simulink library "sm_car_lib_more_examples"  (R2025a)
settings: Solver=VariableStepAuto  StartTime=0.0  StopTime=10.0  RelTol=1e-3
undefined symbols (not defined in the file or in its folder): Linkage, Right, UAc, UAf, UAr, Visual, VisualVisual, X, Y, Z
libraries: sm_lib x109, Suspension_Utilities x45, fl_lib x4, nesl_utility x2
(part 1 of 6)
Description:
  | Copyright 2020-2025 The MathWorks, Inc.
settings Model: Creator=smiller  LastModifiedBy=smiller
settings SolverCC: AlgebraicLoopSolver=TrustRegion
settings DataIOCC: ReturnWorkspaceOutputs=off
settings OptimizationCC: ReuseModelBlockBuffer=off
settings DebuggingCC: UnconnectedInputMsg=warning  UnconnectedOutputMsg=warning  UnconnectedLineMsg=warning  ArithmeticOperatorsInVariantConditions=warning
settings ModelReferenceCC: EnableRefExpFcnMdlSchedulingChecks=on
settings SFSimCC: CustomCodeUndefinedFunction=UseInterfaceOnly
settings RTWCC: GPUComputeCapability=3.5

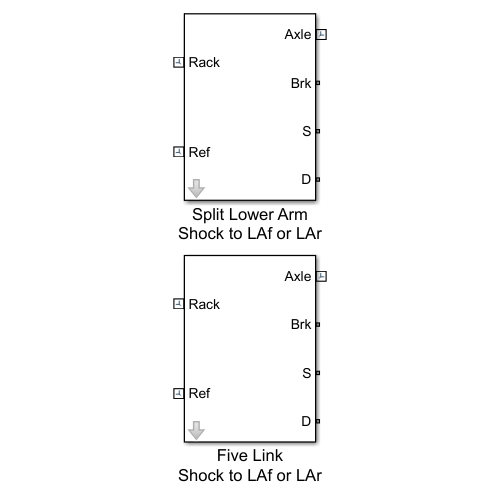
[thumbnail: Simulink's stored preview of the top-level diagram]
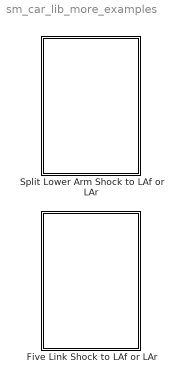
== system sm_car_lib_more_examples ==
  Five Link Shock to LAf or LAr : Subsystem  VariantControl=Link5_StoLAFoR  mask(Five-Link Suspension, Shock to Rear){popup_leftRight=Right, hp_in_f_ua=Linkage.Upper_Arm.HPInboardF.Value, hp_in_r_ua=Linkage.Upper_Arm.HPInboardR.Value, hp_out_f_ua=Linkage.Upper_Arm.HPOutboardF.Value, hp_out_r_ua=Linkage.Upper_Arm.HPOutboardR.Value, hp_in_f_la=Linkage.Lower_Arm.HPInboardF.Value, hp_in_r_la=Linkage.Lower_Arm.HPInboardR.Value, hp_out_f_la=Linkage.Lower_Arm.HPOutboardF.Value, hp_out_r_la=Linkage.Lower_Arm.HPOutboardR.Value, hp_upr_cg=Linkage.Upright.HPCG.Value, hp_upr_wc=Linkage.Upright.HPWheelCtr.Value, hp_in_rod=Linkage.Track_Rod.HPInboard.Value, hp_upr_rod=Linkage.Track_Rod.HPOutboard.Value, hp_spr_top=Linkage.Spring.HPTop.Value, hp_spr_bot=Linkage.Spring.HPBottom.Value, clr_hp=Visual.hp.clr, opc_hp=Visual.hp.opc, size_hp=Visual.hp.rad, uaf_mass=Linkage.Upper_Arm.Mass.Value, uar_mass=Linkage.Upper_Arm.Mass.Value, laf_mass=Linkage.Lower_Arm.Mass.Value, lar_mass=Linkage.Lower_Arm.Mass.Value, clr_conn_links=Visual.hp.clr, opc_conn_links=Visual.hp.opc, size_conn_links=Visual.hp.rad, clr_uaf=Visual.UpperArm.clr, opc_uaf=Visual.part.opc, radius_uaf=Visual.UpperArm.rad, clr_uar=Visual.UpperArm.clr, opc_uar=Visual.part.opc, radius_uar=Visual.UpperArm.rad, clr_laf=Visual.LowerArm.clr, opc_laf=Visual.part.opc, radius_laf=Visual.LowerArm.clr, clr_lar=Visual.LowerArm.clr, opc_lar=Visual.part.opc, radius_lar=Visual.LowerArm.rad, spr_la_att=Linkage.Spring.class.Value, shock_pist_mass=Linkage.Piston.Mass.Value, shock_cyl_mass=Linkage.Cylinder.Mass.Value, up_lim_bumpstop=Linkage.Bumpstops.Upper_Limit.Value, low_lim_bumpstop=Linkage.Bumpstops.Lower_Limit.Value, clr_conn_shock=Visual.hp.clr, opc_conn_shock=Visual.hp.opc, size_conn_shock=Visual.hp.rad, clr_shock_cyl=Visual.Shock.cyl.clr, opc_shock_cyl=Visual.part.opc, radius_shock_cyl=Visual.Shock.cyl.rad, clr_shock_piston=Visual.Shock.piston.clr, opc_shock_piston=Visual.part.opc, clr_shock_bumpstop=Visual.Shock.bumpstop.clr, opc_shock_bumpstop=Visual.part.opc, deadvol_len_shock_cyl=Visual.Shock.dead_length, piston_len_shock=Visual.Shock.piston.len, cyl_cap_len_shock=Visual.Shock.cap.len, bumpstop_len_shock=Visual.Shock.bumpstop.len, atoe=Linkage.Upright.aToe.Value, acamber=Linkage.Upright.aCamber.Value, upr_mass=Linkage.Upright.Mass.Value, clr_conn_upr=Visual.hp.clr, opc_conn_upr=Visual.hp.opc, size_conn_upr=Visual.hp.rad, clr_upr=Visual.Upright.clr, opc_upr=Visual.part.opc, radius_upr=Visual.Upright.clr, clr_stub_axle=Visual.Axle.clr, opc_stub_axle=Visual.part.opc, radius_stub_axle=Visual.Axle.rad, rod_mass=Linkage.Track_Rod.Mass.Value, clr_conn_rod=Visual.hp.clr, opc_conn_rod=Visual.hp.opc, size_conn_rod=Visual.hp.rad, clr_rod=Visual.TrackRod.clr, opc_rod=Visual.part.opc, radius_rod=Visual.TrackRod.rad, whl_spd_init=Linkage.Upright.Initial_Wheel_Speed.Value}
      mask prompts: popup_leftRight "Left/Right"; hp_in_f_ua "Upper Arm Front [xyz] (m)"; hp_in_r_ua "Upper Arm Rear [xyz] (m)"; hp_out_f_ua "Upper Arm Front Outboard [xyz] (m)"; hp_out_r_ua "Upper Arm Rear Outboard [xyz] (m)"; hp_in_f_la "Lower Arm Front [xyz] (m)"; hp_in_r_la "Lower Arm Rear [xyz] (m)"; hp_out_f_la "Lower Arm Front Outboard [xyz] (m)"; hp_out_r_la "Lower Arm Rear Outboard [xyz] (m)"; hp_upr_cg "Upright CG [xyz] (m)"; hp_upr_wc "Wheel Center [xyz] (m)"; hp_in_rod "Track Rod Inboard [xyz] (m)"; hp_upr_rod "Track Rod Outboard [xyz] (m)"; hp_spr_top "Spring Top [xyz] (m)"; hp_spr_bot "Spring Bottom [xyz] (m)"; spr_la_att "Lower Arm Attach (Front/Rear)"; shock_pist_mass "Piston Mass (kg)"; shock_cyl_mass "Cylinder Mass (kg)"; up_lim_bumpstop "Upper Limit (m)"; low_lim_bumpstop "Lower Limit (m)"; deadvol_len_shock_cyl "Dead Volume Height (m)"; piston_len_shock "Piston Length (m)"; cyl_cap_len_shock "Cylinder Cap Length (m)"; bumpstop_len_shock "Bumpstop Length (m)"; atoe "Toe Angle (deg)"; acamber "Camber Angle (deg)"; upr_mass "Mass (kg)"; rod_mass "Mass (kg)"; whl_spd_init "Initial Wheel Speed (rad/s)"
      mask help: This models a multi-link suspension for steered and non-steered configurations. The non-steered configuration maintains its orientation via the track rods that connect to fixed points on the subframe. The shock absorber connects the subframe and lower rear control arm.
      mask init:
      | if(popup_leftRight == 1)
      |     rhs_susp = 1;
      |     set_param([gcb '/Spring Arm/Front/Arm'],'popup_leftRight','Left');
      |     set_param([gcb '/Spring Arm/Rear/Arm'],'popup_leftRight','Left');
      | elseif(popup_leftRight == 2)
      |     rhs_susp = -1;
      |     set_param([gcb '/Spring Arm/Front/Arm'],'popup_leftRight','Right');
      |     set_param([gcb '/Spring Arm/Rear/Arm'],'popup_leftRight','Right');
      | end
      | 
      | if(strcmpi(spr_la_att,'front'))
      |     set_param([gcb '/Spring Arm'],'LabelModeActiveChoice','Front');
      | elseif(strcmpi(spr_la_att,'rear'))
      |     set_param([gcb '/Spring Arm'],'LabelModeActiveChoice','Rear');
      | end
      mask Help: web('sm_car_double_wishbone_suspension_help.html')
      mask TypeOptions popup_leftRight:
      | Hardpoints/popup_leftRight | Upright/popup_leftRight | Lower Arm Rear/popup_leftRight | Lower Arm Front/popup_leftRight | Track Rod/popup_leftRight | Upper Arm Front/popup_leftRight | Upper Arm Rear/popup_leftRight | Universal
      | HP LAF/popup_leftRight | Universal
      | HP LAR/popup_leftRight | Universal
      | HP UAF/popup_leftRight | Universal
      | HP UAR/popup_leftRight
      mask TypeOptions hp_in_f_ua:
      | Hardpoints/hp_in_f_ua | Upper Arm Front/hp_in | Universal
      | HP UAF/hp_f | Universal
      | HP UAR/hp_f
      mask TypeOptions hp_in_r_ua:
      | Hardpoints/hp_in_r_ua | Upper Arm Rear/hp_in | Universal
      | HP UAF/hp_r | Universal
      | HP UAR/hp_r
      mask TypeOptions hp_out_f_ua: Upper Arm Front/hp_out | Upright/hp_uaf_out
      mask TypeOptions hp_out_r_ua: Upper Arm Rear/hp_out | Upright/hp_uar_out
      mask TypeOptions hp_in_f_la:
      | Hardpoints/hp_in_f_la | Lower Arm Front/hp_in | Universal
      | HP LAF/hp_f | Universal
      | HP LAR/hp_f
      mask TypeOptions hp_in_r_la:
      | Hardpoints/hp_in_r_la | Lower Arm Rear/hp_in | Universal
      | HP LAF/hp_r | Universal
      | HP LAR/hp_r
      mask TypeOptions hp_out_f_la: Upright/hp_laf_out | Lower Arm Front/hp_out
      mask TypeOptions hp_out_r_la: Upright/hp_lar_out | Lower Arm Rear/hp_out
      mask TypeOptions hp_upr_cg: Upright/hp_upr_cg
      mask TypeOptions hp_upr_wc: Upright/hp_upr_wc
      mask TypeOptions hp_in_rod: Track Rod/hp_in
      mask TypeOptions hp_upr_rod: Track Rod/hp_out | Upright/hp_upr_rod
      mask TypeOptions hp_spr_top: Hardpoints/hp_spr_top | Shock Absorber/hp_spr_top
      mask TypeOptions hp_spr_bot: Shock Absorber/hp_spr_bot | Lower Arm Rear/hp_spr
      mask TypeOptions clr_hp: Hardpoints/clr_hp
      mask TypeOptions opc_hp: Hardpoints/opc_hp
      mask TypeOptions size_hp: Hardpoints/size_hp
      mask TypeOptions uaf_mass: Upper Arm Front/rod_mass
      mask TypeOptions uar_mass: Upper Arm Rear/rod_mass
      mask TypeOptions laf_mass: Lower Arm Front/rod_mass
      mask TypeOptions lar_mass: Lower Arm Rear/rod_mass
      mask TypeOptions clr_conn_links: Upper Arm Front/clr_conn_rod | Upper Arm Rear/clr_conn_rod | Lower Arm Front/clr_conn_rod | Lower Arm Rear/clr_conn_rod
      mask TypeOptions opc_conn_links: Upper Arm Front/opc_conn_rod | Upper Arm Rear/opc_conn_rod | Lower Arm Front/opc_conn_rod | Lower Arm Rear/opc_conn_rod
      mask TypeOptions size_conn_links: Upper Arm Front/size_conn_rod | Upper Arm Rear/size_conn_rod | Lower Arm Front/size_conn_rod | Lower Arm Rear/size_conn_rod
      mask TypeOptions clr_uaf: Upper Arm Front/clr_rod
      mask TypeOptions opc_uaf: Upper Arm Front/opc_rod
      mask TypeOptions radius_uaf: Upper Arm Front/radius_rod
      mask TypeOptions clr_uar: Upper Arm Rear/clr_rod
      mask TypeOptions opc_uar: Upper Arm Rear/opc_rod
      mask TypeOptions radius_uar: Upper Arm Rear/radius_rod
      mask TypeOptions clr_laf: Lower Arm Rear/clr_rod
      mask TypeOptions opc_laf: Lower Arm Rear/opc_rod
      mask TypeOptions radius_laf: Lower Arm Rear/radius_rod
      mask TypeOptions clr_lar: Lower Arm Front/clr_rod
      mask TypeOptions opc_lar: Lower Arm Front/opc_rod
      mask TypeOptions radius_lar: Lower Arm Front/radius_rod
      mask TypeOptions shock_pist_mass: Shock Absorber/shock_pist_mass
      mask TypeOptions shock_cyl_mass: Shock Absorber/shock_cyl_mass
      mask TypeOptions up_lim_bumpstop: Shock Absorber/up_lim_bumpstop
      mask TypeOptions low_lim_bumpstop: Shock Absorber/low_lim_bumpstop
      mask TypeOptions clr_conn_shock: Shock Absorber/clr_conn_shock
      mask TypeOptions opc_conn_shock: Shock Absorber/opc_conn_shock
      mask TypeOptions size_conn_shock: Shock Absorber/size_conn_shock
      mask TypeOptions clr_shock_cyl: Shock Absorber/clr_shock_cyl
      mask TypeOptions opc_shock_cyl: Shock Absorber/opc_shock_cyl
      mask TypeOptions radius_shock_cyl: Shock Absorber/radius_shock_cyl
      mask TypeOptions clr_shock_piston: Shock Absorber/clr_shock_piston
      mask TypeOptions opc_shock_piston: Shock Absorber/opc_shock_piston
      mask TypeOptions clr_shock_bumpstop: Shock Absorber/clr_shock_bumpstop
      mask TypeOptions opc_shock_bumpstop: Shock Absorber/opc_shock_bumpstop
      mask TypeOptions deadvol_len_shock_cyl: Shock Absorber/deadvol_len_shock_cyl
      mask TypeOptions piston_len_shock: Shock Absorber/piston_len_shock
      mask TypeOptions cyl_cap_len_shock: Shock Absorber/cyl_cap_len_shock
      mask TypeOptions bumpstop_len_shock: Shock Absorber/bumpstop_len_shock
      mask TypeOptions atoe: Upright/atoe
      mask TypeOptions acamber: Upright/acamber
      mask TypeOptions upr_mass: Upright/upr_mass
      mask TypeOptions clr_conn_upr: Upright/clr_conn_upr
      mask TypeOptions opc_conn_upr: Upright/opc_conn_upr
      mask TypeOptions size_conn_upr: Upright/size_conn_upr
      mask TypeOptions clr_upr: Upright/clr_upr
      mask TypeOptions opc_upr: Upright/opc_upr
      mask TypeOptions radius_upr: Upright/radius_upr
      mask TypeOptions clr_stub_axle: Upright/clr_stub_axle
      mask TypeOptions opc_stub_axle: Upright/opc_stub_axle
      mask TypeOptions radius_stub_axle: Upright/radius_stub_axle
      mask TypeOptions rod_mass: Track Rod/rod_mass
      mask TypeOptions clr_conn_rod: Track Rod/clr_conn_rod
      mask TypeOptions opc_conn_rod: Track Rod/opc_conn_rod
      mask TypeOptions size_conn_rod: Track Rod/size_conn_rod
      mask TypeOptions clr_rod: Track Rod/clr_rod
      mask TypeOptions opc_rod: Track Rod/opc_rod
      mask TypeOptions radius_rod: Track Rod/radius_rod
      mask TypeOptions whl_spd_init: Upright/whl_spd_init
      mask DialogControl cont_hp Prompt: Hardpoints
      mask DialogControl cont_vis_hp Prompt: Visualization
      mask DialogControl text_clr_hp Prompt: Color [RGB]
      mask DialogControl text_opc_hp Prompt: Opac. (0-1)
      mask DialogControl text_size_hp Prompt: Size (m)
      mask DialogControl text_hp Prompt: Hardpoints
      mask DialogControl cont_links Prompt: Links
      mask DialogControl text_links_part Prompt: Part
      mask DialogControl text_links_mass Prompt: Mass (kg)
      mask DialogControl text_upper_f Prompt: Upper, Front
      mask DialogControl text_upper_r Prompt: Upper, Rear
      mask DialogControl text_lower_f Prompt: Lower, Front
      mask DialogControl text_lower_r Prompt: Lower, Rear
      mask DialogControl cont_vis_links Prompt: Visualization
      mask DialogControl text_vis_links_clr Prompt: Color [RGB]
      mask DialogControl text_vis_links_opc Prompt: Opacity (0-1)
      mask DialogControl text_vis_links_rad Prompt: Radius (m)
      mask DialogControl text_vis_links_conn Prompt: Connections
      mask DialogControl text_vis_links_uaf Prompt: Upper, Front
      mask DialogControl text_vis_links_uar Prompt: Upper, Rear
      mask DialogControl text_vis_links_laf Prompt: Lower, Front
      mask DialogControl text_vis_links_lar Prompt: Lower, Rear
      mask DialogControl cont_shock Prompt: Shock
      mask DialogControl cont_parts Prompt: Parts
      mask DialogControl cont_bumpstop Prompt: Bumpstop
      mask DialogControl cont_vis_shock Prompt: Visualization
      mask DialogControl text_clr_shock Prompt: Color  [RGB]
      mask DialogControl text_opc_shock Prompt: Opac. (0-1)
      mask DialogControl text_size_shock Prompt: Size (m)
      mask DialogControl text_conn_shock Prompt: Connections
      mask DialogControl text_shock_shock Prompt: Cylinder
      mask DialogControl text_shock_piston Prompt: Piston
      mask DialogControl text_piston_radius Prompt: <cylinder radius>
      mask DialogControl text_shock_bumpstop Prompt: Bumpstop
      mask DialogControl text_bumpstop_radius Prompt: <cylinder radius>
      mask DialogControl cont_upright Prompt: Upright
      mask DialogControl grp_upright Prompt: Upright
      mask DialogControl cont_vis_upr Prompt: Visualization
      mask DialogControl text_clr_upr Prompt: Color [RGB]
      mask DialogControl text_opc_upr Prompt: Opac. (0-1)
      mask DialogControl text_size_upr Prompt: Size (m)
      mask DialogControl text_conn_upr Prompt: Connections
      mask DialogControl text_upright Prompt: Upright
      mask DialogControl text_stub_axle Prompt: Stub Axle
      mask DialogControl cont_steer Prompt: Steer
      mask DialogControl grp_rod Prompt: Rod
      mask DialogControl cont_vis_rod Prompt: Visualization
      mask DialogControl text_clr_rod Prompt: Color [RGB]
      mask DialogControl text_opc_rod Prompt: Opac. (0-1)
      mask DialogControl text_size_rod Prompt: Size (m)
      mask DialogControl text_conn_rod Prompt: Connections
      mask DialogControl text_rod_rod Prompt: Rod
      mask DialogControl cont_initial Prompt: Initial
  Split Lower Arm Shock to LAf or LAr : Subsystem  VariantControl=SplitLA_StoLAFoR  mask(Double-Wishbone Suspension B){popup_leftRight=Right, hp_in_f_ua=Linkage.Upper_Arm.HPInboardF.Value, hp_in_r_ua=Linkage.Upper_Arm.HPInboardR.Value, hp_out_ua=Linkage.Upper_Arm.HPOutboard.Value, hp_in_f_la=Linkage.Lower_Arm.HPInboardF.Value, hp_in_r_la=Linkage.Lower_Arm.HPInboardR.Value, hp_out_f_la=Linkage.Lower_Arm.HPOutboardF.Value, hp_out_r_la=Linkage.Lower_Arm.HPOutboardR.Value, hp_upr_cg=Linkage.Upright.HPCG.Value, hp_upr_wc=Linkage.Upright.HPWheelCtr.Value, hp_in_rod=Linkage.Track_Rod.HPInboard.Value, hp_upr_rod=Linkage.Track_Rod.HPOutboard.Value, hp_spr_top=Linkage.Spring.HPTop.Value, hp_spr_bot=Linkage.Spring.HPBottom.Value, clr_hp=Visual.hp.clr, opc_hp=Visual.hp.opc, size_hp=Visual.hp.rad, popup_conn_ua=One Rigid, ua_mass=Linkage.Upper_Arm.Mass.Value, clr_ua=Visual.UpperArm.clr, opc_ua=Visual.part.opc, radius_ua=Visual.UpperArm.rad, laf_mass=Linkage.Lower_Arm.Mass.Value, lar_mass=Linkage.Lower_Arm.Mass.Value, clr_conn_la=Visual.hp.clr, opc_conn_la=Visual.hp.opc, size_conn_la=VisualVisual.hp.rad, clr_laf=Visual.LowerArm.clr, opc_laf=Visual.part.opc, radius_laf=Visual.LowerArm.rad, clr_lar=Visual.LowerArm.clr, opc_lar=VisualVisual.part.opc, radius_lar=Visual.LowerArm.rad, spr_la_att=Linkage.Spring.class.Value, shock_pist_mass=Linkage.Piston.Mass.Value, shock_cyl_mass=Linkage.Cylinder.Mass.Value, up_lim_bumpstop=Linkage.Bumpstops.Upper_Limit.Value, low_lim_bumpstop=Linkage.Bumpstops.Lower_Limit.Value, clr_conn_shock=Visual.hp.clr, opc_conn_shock=Visual.hp.opc, size_conn_shock=Visual.hp.rad, clr_shock_cyl=Visual.Shock.cyl.clr, opc_shock_cyl=Visual.part.opc, radius_shock_cyl=Visual.Shock.cyl.rad, clr_shock_piston=Visual.Shock.piston.clr, opc_shock_piston=Visual.part.opc, clr_shock_bumpstop=Visual.Shock.bumpstop.clr, opc_shock_bumpstop=Visual.part.opc, deadvol_len_shock_cyl=Visual.Shock.dead_length, piston_len_shock=Visual.Shock.piston.len, cyl_cap_len_shock=Visual.Shock.cap.len, bumpstop_len_shock=Visual.Shock.bumpstop.len, atoe=Linkage.Upright.aToe.Value, acamber=Linkage.Upright.aCamber.Value, upr_mass=Linkage.Upright.Mass.Value, clr_conn_upr=Visual.hp.clr, opc_conn_upr=Visual.hp.opc, size_conn_upr=Visual.hp.rad, clr_upr=Visual.Upright.clr, opc_upr=Visual.part.opc, radius_upr=Visual.Upright.rad, clr_stub_axle=Visual.Axle.clr, opc_stub_axle=Visual.part.opc, radius_stub_axle=Visual.Axle.rad, rod_mass=Linkage.Track_Rod.Mass.Value, clr_conn_rod=Visual.hp.clr, opc_conn_rod=Visual.hp.opc, size_conn_rod=Visual.hp.rad, clr_rod=Visual.TrackRod.clr, opc_rod=Visual.part.opc, radius_rod=Visual.TrackRod.rad, whl_spd_init=Linkage.Upright.Initial_Wheel_Speed.Value}
      mask prompts: popup_leftRight "Left/Right"; hp_in_f_ua "Upper Arm Front [xyz] (m)"; hp_in_r_ua "Upper Arm Rear [xyz] (m)"; hp_out_ua "Upper Arm Outboard [xyz] (m)"; hp_in_f_la "Lower Arm Front [xyz] (m)"; hp_in_r_la "Lower Arm Rear [xyz] (m)"; hp_out_f_la "Lower Arm Front Outboard [xyz] (m)"; hp_out_r_la "Lower Arm Rear Outboard [xyz] (m)"; hp_upr_cg "Upright CG [xyz] (m)"; hp_upr_wc "Wheel Center [xyz] (m)"; hp_in_rod "Track Rod Inboard [xyz] (m)"; hp_upr_rod "Track Rod Outboard [xyz] (m)"; hp_spr_top "Spring Top [xyz] (m)"; hp_spr_bot "Spring Bottom [xyz] (m)"; popup_conn_ua "Subframe Connection"; ua_mass "Mass (kg)"; clr_ua "Color [RGB]"; opc_ua "Opacity (0-1)"; radius_ua "Radius (m)"; spr_la_att "Lower Arm Attach (Front/Rear)"; shock_pist_mass "Piston Mass (kg)"; shock_cyl_mass "Cylinder Mass (kg)"; up_lim_bumpstop "Upper Limit (m)"; low_lim_bumpstop "Lower Limit (m)"; deadvol_len_shock_cyl "Dead Volume Height (m)"; piston_len_shock "Piston Length (m)"; cyl_cap_len_shock "Cylinder Cap Length (m)"; bumpstop_len_shock "Bumpstop Length (m)"; atoe "Toe Angle (deg)"; acamber "Camber Angle (deg)"; upr_mass "Mass (kg)"; rod_mass "Mass (kg)"; whl_spd_init "Initial Wheel Speed (rad/s)"
      mask help:
      | This models a double-wishbone suspension for steered and non-steered configurations.  The non-steered configuration maintains its orientation via the track rods that connect to fixed points on the subframe.
      |
      | This version contains a new implementation for the upright that defaults to zero toe and zero camber, regardless of hardpoint positions (still testing).
      mask init:
      | if(popup_leftRight == 1)
      |     rhs_susp = 1;
      |     set_param([gcb '/Spring Arm/Front/Arm'],'popup_leftRight','Left');
      |     set_param([gcb '/Spring Arm/Rear/Arm'],'popup_leftRight','Left');
      | elseif(popup_leftRight == 2)
      |     rhs_susp = -1;
      |     set_param([gcb '/Spring Arm/Front/Arm'],'popup_leftRight','Right');
      |     set_param([gcb '/Spring Arm/Rear/Arm'],'popup_leftRight','Right');
      | end
      | 
      | if(popup_conn_ua == 1)
      |     set_param([gcb '/HP UA'],'OverrideUsingVariant','Rigid_1Rev');
      | elseif(popup_conn_ua == 2)
      |     set_param([gcb '/HP UA'],'OverrideUsingVariant','Rigid_2Rev');
      | elseif(popup_conn_ua == 3)
      |     set_param([gcb '/HP UA'],'OverrideUsingVariant','Bushings');
      | end
      | 
      | if(strcmpi(spr_la_att,'front'))
      |     set_param([gcb '/Spring Arm'],'LabelModeActiveChoice','Front');
      | elseif(strcmpi(spr_la_att,'rear'))
      |     set_param([gcb '/Spring Arm'],'LabelModeActiveChoice','Rear');
      | end
      mask Help: web('sm_car_double_wishbone_suspension_help.html')
      mask TypeOptions popup_leftRight:
      | Hardpoints/popup_leftRight | Upper Arm/popup_leftRight | Upright/popup_leftRight | Lower Arm Front/popup_leftRight | Lower Arm Rear/popup_leftRight | Track Rod/popup_leftRight | Universal
      | HP LAF/popup_leftRight | Universal
      | HP LAR/popup_leftRight
      mask TypeOptions hp_in_f_ua: Upper Arm/hp_in_f | Hardpoints/hp_in_f_ua
      mask TypeOptions hp_in_r_ua: Upper Arm/hp_in_r | Hardpoints/hp_in_r_ua
      mask TypeOptions hp_out_ua: Upper Arm/hp_out | Upright/hp_ua_out
      mask TypeOptions hp_in_f_la:
      | Hardpoints/hp_in_f_la | Lower Arm Front/hp_in | Universal
      | HP LAF/hp_f | Universal
      | HP LAR/hp_f
      mask TypeOptions hp_in_r_la:
      | Hardpoints/hp_in_r_la | Lower Arm Rear/hp_in | Universal
      | HP LAF/hp_r | Universal
      | HP LAR/hp_r
      mask TypeOptions hp_out_f_la: Upright/hp_laf_out | Lower Arm Front/hp_out
      mask TypeOptions hp_out_r_la: Upright/hp_lar_out | Lower Arm Rear/hp_out
      mask TypeOptions hp_upr_cg: Upright/hp_upr_cg
      mask TypeOptions hp_upr_wc: Upright/hp_upr_wc
      mask TypeOptions hp_in_rod: Track Rod/hp_in
      mask TypeOptions hp_upr_rod: Track Rod/hp_out | Upright/hp_upr_rod
      mask TypeOptions hp_spr_top: Hardpoints/hp_spr_top | Shock Absorber/hp_spr_top
      mask TypeOptions hp_spr_bot: Shock Absorber/hp_spr_bot | Lower Arm Front/hp_spr
      mask TypeOptions clr_hp: Hardpoints/clr_hp
      mask TypeOptions opc_hp: Hardpoints/opc_hp
      mask TypeOptions size_hp: Hardpoints/size_hp
      mask TypeOptions popup_conn_ua: One Rigid | Two Rigid | Two Bushings
      mask TypeOptions ua_mass: Upper Arm/ua_mass
      mask TypeOptions clr_ua: Upper Arm/clr_ua
      mask TypeOptions opc_ua: Upper Arm/opc_ua
      mask TypeOptions radius_ua: Upper Arm/radius_ua
      mask TypeOptions laf_mass: Front Arm to Spring/Front/Arm /rod_mass
      mask TypeOptions lar_mass: Lower Arm Rear/rod_mass
      mask TypeOptions clr_conn_la: Front Arm to Spring/Front/Arm /clr_conn_rod | Lower Arm Rear/clr_conn_rod
      mask TypeOptions opc_conn_la: Front Arm to Spring/Front/Arm /opc_conn_rod | Lower Arm Rear/opc_conn_rod
      mask TypeOptions size_conn_la: Front Arm to Spring/Front/Arm /size_conn_rod | Lower Arm Rear/size_conn_rod
      mask TypeOptions clr_laf: Lower Arm Rear/clr_rod
      mask TypeOptions opc_laf: Lower Arm Rear/opc_rod
      mask TypeOptions radius_laf: Lower Arm Rear/radius_rod
      mask TypeOptions clr_lar: Front Arm to Spring/Front/Arm /clr_rod
      mask TypeOptions opc_lar: Front Arm to Spring/Front/Arm /opc_rod
      mask TypeOptions radius_lar: Front Arm to Spring/Front/Arm /radius_rod
      mask TypeOptions shock_pist_mass: Shock Absorber/shock_pist_mass
      mask TypeOptions shock_cyl_mass: Shock Absorber/shock_cyl_mass
      mask TypeOptions up_lim_bumpstop: Shock Absorber/up_lim_bumpstop
      mask TypeOptions low_lim_bumpstop: Shock Absorber/low_lim_bumpstop
      mask TypeOptions clr_conn_shock: Shock Absorber/clr_conn_shock
      mask TypeOptions opc_conn_shock: Shock Absorber/opc_conn_shock
      mask TypeOptions size_conn_shock: Shock Absorber/size_conn_shock
      mask TypeOptions clr_shock_cyl: Shock Absorber/clr_shock_cyl
      mask TypeOptions opc_shock_cyl: Shock Absorber/opc_shock_cyl
      mask TypeOptions radius_shock_cyl: Shock Absorber/radius_shock_cyl
      mask TypeOptions clr_shock_piston: Shock Absorber/clr_shock_piston
      mask TypeOptions opc_shock_piston: Shock Absorber/opc_shock_piston
      mask TypeOptions clr_shock_bumpstop: Shock Absorber/clr_shock_bumpstop
      mask TypeOptions opc_shock_bumpstop: Shock Absorber/opc_shock_bumpstop
      mask TypeOptions deadvol_len_shock_cyl: Shock Absorber/deadvol_len_shock_cyl
      mask TypeOptions piston_len_shock: Shock Absorber/piston_len_shock
      mask TypeOptions cyl_cap_len_shock: Shock Absorber/cyl_cap_len_shock
      mask TypeOptions bumpstop_len_shock: Shock Absorber/bumpstop_len_shock
      mask TypeOptions atoe: Upright/atoe
      mask TypeOptions acamber: Upright/acamber
      mask TypeOptions upr_mass: Upright/upr_mass
      mask TypeOptions clr_conn_upr: Upright/clr_conn_upr
      mask TypeOptions opc_conn_upr: Upright/opc_conn_upr
      mask TypeOptions size_conn_upr: Upright/size_conn_upr
      mask TypeOptions clr_upr: Upright/clr_upr
      mask TypeOptions opc_upr: Upright/opc_upr
      mask TypeOptions radius_upr: Upright/radius_upr
      mask TypeOptions clr_stub_axle: Upright/clr_stub_axle
      mask TypeOptions opc_stub_axle: Upright/opc_stub_axle
      mask TypeOptions radius_stub_axle: Upright/radius_stub_axle
      mask TypeOptions rod_mass: Track Rod/rod_mass
      mask TypeOptions clr_conn_rod: Track Rod/clr_conn_rod
      mask TypeOptions opc_conn_rod: Track Rod/opc_conn_rod
      mask TypeOptions size_conn_rod: Track Rod/size_conn_rod
      mask TypeOptions clr_rod: Track Rod/clr_rod
      mask TypeOptions opc_rod: Track Rod/opc_rod
      mask TypeOptions radius_rod: Track Rod/radius_rod
      mask TypeOptions whl_spd_init: Upright/whl_spd_init
      mask DialogControl cont_hp Prompt: Hardpoints
      mask DialogControl cont_vis_hp Prompt: Visualization
      mask DialogControl text_clr_hp Prompt: Color [RGB]
      mask DialogControl text_opc_hp Prompt: Opac. (0-1)
      mask DialogControl text_size_hp Prompt: Size (m)
      mask DialogControl text_hp Prompt: Hardpoints
      mask DialogControl cont_ua Prompt: UA
      mask DialogControl cont_vis_ua Prompt: Visualization
      mask DialogControl cont_laf Prompt: LA
      mask DialogControl text_la_part Prompt: Part
      mask DialogControl text_la_mass Prompt: Mass (kg)
      mask DialogControl text_la_front Prompt: Lower, Front
      mask DialogControl text_la_rear Prompt: Lower, Rear
      mask DialogControl cont_vis_laf Prompt: Visualization
      mask DialogControl text_vis_la_clr Prompt: Color [RGB]
      mask DialogControl text_vis_la_opc Prompt: Opacity (0-1)
      mask DialogControl text_vis_la_rad Prompt: Radius (m)
      mask DialogControl text_vis_la_hp Prompt: Hardpoints
      mask DialogControl text_vis_la_f Prompt: Lower, Front
      mask DialogControl text_vis_la_r Prompt: Lower, Rear
      mask DialogControl cont_shock Prompt: Shock
      mask DialogControl cont_parts Prompt: Parts
      mask DialogControl cont_bumpstop Prompt: Bumpstop
      mask DialogControl cont_vis_shock Prompt: Visualization
      mask DialogControl text_clr_shock Prompt: Color  [RGB]
      mask DialogControl text_opc_shock Prompt: Opac. (0-1)
      mask DialogControl text_size_shock Prompt: Size (m)
      mask DialogControl text_conn_shock Prompt: Connections
      mask DialogControl text_shock_shock Prompt: Cylinder
      mask DialogControl text_shock_piston Prompt: Piston
      mask DialogControl text_piston_radius Prompt: <cylinder radius>
      mask DialogControl text_shock_bumpstop Prompt: Bumpstop
      mask DialogControl text_bumpstop_radius Prompt: <cylinder radius>
      mask DialogControl cont_upright Prompt: Upright
      mask DialogControl grp_upright Prompt: Upright
      mask DialogControl cont_vis_upr Prompt: Visualization
      mask DialogControl text_clr_upr Prompt: Color [RGB]
      mask DialogControl text_opc_upr Prompt: Opac. (0-1)
      mask DialogControl text_size_upr Prompt: Size (m)
      mask DialogControl text_conn_upr Prompt: Connections
      mask DialogControl text_upright Prompt: Upright
      mask DialogControl text_stub_axle Prompt: Stub Axle
      mask DialogControl cont_steer Prompt: Steer
      mask DialogControl grp_rod Prompt: Rod
      mask DialogControl cont_vis_rod Prompt: Visualization
      mask DialogControl text_clr_rod Prompt: Color [RGB]
      mask DialogControl text_opc_rod Prompt: Opac. (0-1)
      mask DialogControl text_size_rod Prompt: Size (m)
      mask DialogControl text_conn_rod Prompt: Connections
      mask DialogControl text_rod_rod Prompt: Rod
      mask DialogControl cont_initial Prompt: Initial
